simulink model "a1ae2(2)"  (R2022a)
settings: Solver=VariableStepAuto  StartTime=0.0  StopTime=1000  MaxStep=0.1  RelTol=1e-3
settings Model: Creator=attit  LastModifiedBy=attit
settings DataIOCC: ReturnWorkspaceOutputs=off

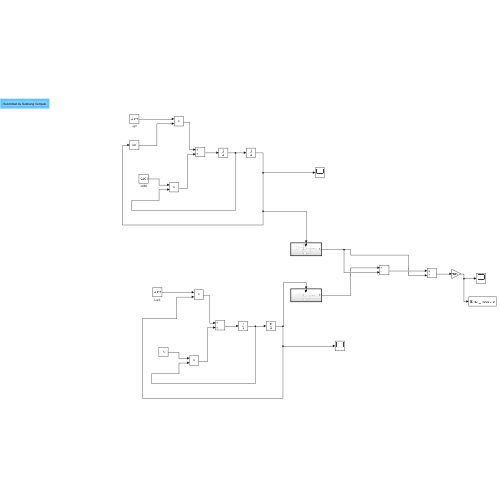
[thumbnail: Simulink's stored preview of the top-level diagram]
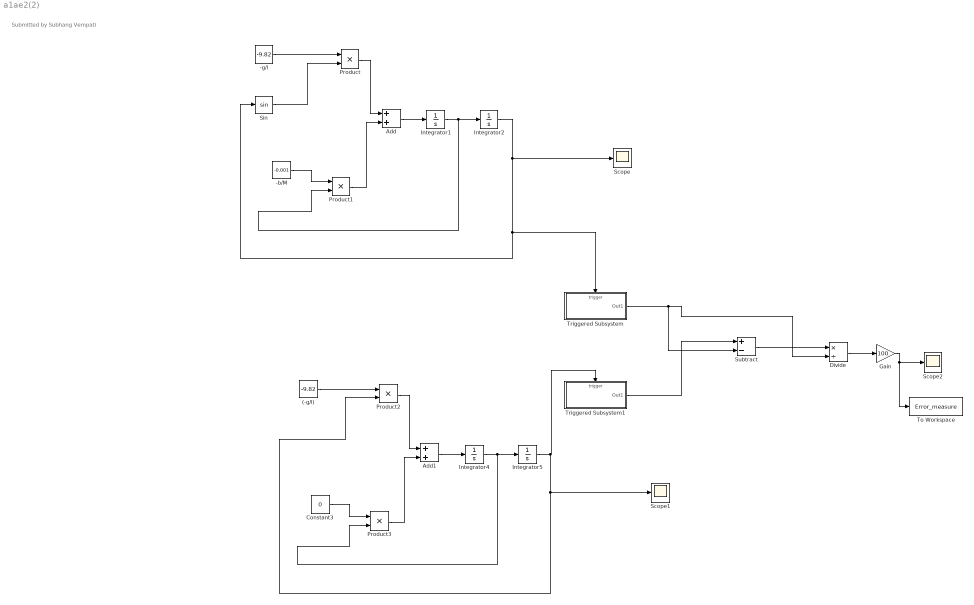
== system a1ae2(2) ==
  note: Submitted by Subhang Vempati
  (-g/l) : Constant  Value=-9.82
  -b/M : Constant  Value=-0.001
  -g/l : Constant  Value=-9.82
  Add : Sum
  Add1 : Sum
  Constant3 : Constant  Value=0
  Divide : Product  Inputs=*/
  Gain : Gain  Gain=100
  Integrator1 : Integrator
  Integrator2 : Integrator  InitialCondition=pi/4
  Integrator4 : Integrator
  Integrator5 : Integrator  InitialCondition=pi/4
  Product{,1..3} (4 alike) : Product
  Scope : Scope
  Scope1 : Scope
  Scope2 : Scope
  Sin : Trigonometry
  Subtract : Sum  Inputs=+-
  To Workspace : ToWorkspace  VariableName=Error_measure  SaveFormat=Timeseries  SampleTime=-1
  Triggered Subsystem : Subsystem  TreatAsAtomicUnit=on
  Triggered Subsystem1 : Subsystem  TreatAsAtomicUnit=on
  wires:
  Integrator1/1 -> Product1/2, Integrator2/1
  Integrator2/1 -> Triggered Subsystem/Trigger, Sin/1, Scope/1
  Sin/1 -> Product/2
  Add/1 -> Integrator1/1
  -g/l/1 -> Product/1
  Product/1 -> Add/1
  Product1/1 -> Add/2
  -b/M/1 -> Product1/1
  Integrator4/1 -> Product3/2, Integrator5/1
  Integrator5/1 -> Triggered Subsystem1/Trigger, Product2/2, Scope1/1
  Add1/1 -> Integrator4/1
  (-g/l)/1 -> Product2/1
  Product2/1 -> Add1/1
  Product3/1 -> Add1/2
  Constant3/1 -> Product3/1
  Triggered Subsystem/1(Out1) -> Subtract/2, Divide/2
  Subtract/1 -> Divide/1
  Divide/1 -> Gain/1
  Gain/1 -> Scope2/1, To Workspace/1
  Triggered Subsystem1/1(Out1) -> Subtract/1

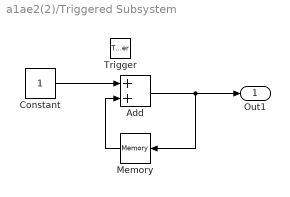
== system a1ae2(2)/Triggered Subsystem ==
  Trigger : TriggerPort  VariantControl=(inherit)
  Add : Sum
  Constant : Constant
  Memory : Memory  InheritSampleTime=on
  Out1 : Outport
  wires:
  Constant/1 -> Add/1
  Add/1 -> Memory/1, Out1/1
  Memory/1 -> Add/2

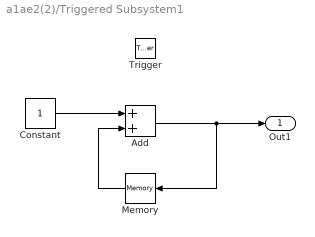
== system a1ae2(2)/Triggered Subsystem1 ==
  Trigger : TriggerPort  VariantControl=(inherit)
  Add : Sum
  Constant : Constant
  Memory : Memory  InheritSampleTime=on
  Out1 : Outport
  wires:
  Constant/1 -> Add/1
  Memory/1 -> Add/2
  Add/1 -> Memory/1, Out1/1
